simulink model "flightControlSystem"  (R2022b)
settings: Solver=ode3  StartTime=0  StopTime=TFinal  FixedStep=Ts  RelTol=1e-3  EnableMultiTasking=on
undefined symbols (not defined in the file): codertarget, Controller, DiscIntNeverNeededParam, Discrete, Estimator, g, init, orient_ref, pos_ref, Sensors, Time, Ts, var_acc_angle_N, var_bias_gyr_N, var_gyro_p_N, Vehicle
libraries: simulink x52, matrix_library x15, slpidlib x4, ctrlSharedLib x4, sharedtransform x3, visiontransforms x2, dspindex x2, visiontextngfix x1, visionanalysis x1, visionstatistics x1, parrotlib x1
(part 3 of 3)

== system flightControlSystem/Control System/State Estimator/XY Position Estimator/EstimatorVelocity/xy velocity w//o angular velocity compensation ==
  note: Optical flow raw readings are converted to velocity in m/s based on the estimated altitude
  optical_flow : Inport
  z_estimate : Inport  Port=2
  " " : Product  Inputs=**
  Compare To Constant : simulink/Logic and Bit Operations/Compare To Constant  relop=<  const=200*4  OutDataTypeStr=boolean
  Counter Free-Running : simulink/Sources/Counter Free-Running  NumBits=32  tsamp=-1
  Gain : Gain  Gain=-1
  Select dxy : Selector  InputPortWidth=3  IndexOptions=Index vector (dialog)  Indices=[1 2]  OutputSizes=1
  Switch : Switch  Criteria=u2 > Threshold  SaturateOnIntegerOverflow=off  InputSameDT=off
  opticalFlowErrorCorrect : Gain  Gain=1.15
  optical_flow_dx_dy : Outport
  wires:
  Select dxy/1 -> optical_flow_dx_dy/1  "optical_flow_dx_dy"
  " "/1 -> opticalFlowErrorCorrect/1
  opticalFlowErrorCorrect/1 -> Switch/3
  Gain/1 -> " "/2
  Switch/1 -> Select dxy/1
  Counter Free-Running/1 -> Compare To Constant/1
  Compare To Constant/1 -> Switch/2
  optical_flow/1 -> " "/1, Switch/1
  z_estimate/1 -> Gain/1

== matlab function flightControlSystem/Control System/Controller/Position Controller/Position error transformation (Earth to Body frame) ==
  data: yaw input; xy_err_earth input; xy_err_body output
function xy_err_body = fcn(yaw,xy_err_earth)

transformation = [cos(yaw), sin(yaw); -sin(yaw),  cos(yaw)];
xy_err_body = transformation * xy_err_earth;


end

== matlab function flightControlSystem/Image Processing System/Find Angle of a Turn ==
  data: lines input; alpha output; right input; left input
function alpha = getAlpha(lines, right, left)
if right==1 || left==1
    if lines
        %lines(1,1) -- point1.col
        %lines(1,2) -- point1.row
        %lines(1,3) -- point2.col
        %lines(1,4) -- point2.row
        l = double(abs(lines(1,3)-lines(1,1)));
        d = sqrt(double((lines(1,1)-lines(1,3))^2+(lines(1,2)-lines(1,4))^2));
        alpha = acos(l/d);
        
        %Ignore short edge
        if d >= 20
            if right==1
                if (lines(1,2) > lines(1,4) && lines(1,1) <= lines(1,3))||(lines(1,2) < lines(1,4) && lines(1,1) > lines(1,3))
                    alpha = -alpha;
                end
            else
                if (lines(1,2) < lines(1,4) && lines(1,1) <= lines(1,3))||(lines(1,2) > lines(1,4) && lines(1,1) > lines(1,3))
                    alpha = -alpha;
                end
            end
    
            alpha = pi/2 + alpha;
        else
            alpha = 0;
        end
    else
        alpha = 0;
    end
else
    alpha = 0;
end

== stateflow chart flightControlSystem/Control System/Path Planning/Chart ==
  state AlignRight
    during:
    xOut = xOut - 0.0005*sin(yaw_est);
    yOut = yOut + 0.0005*cos(yaw_est);
  state AlignLeft
    during:
    xOut = xOut + 0.0005*sin(yaw_est);
    yOut = yOut - 0.0005*cos(yaw_est);
  state MoveToTargetYawRight
    entry:
    doState = 0;
    during:
    if (doState==0)
    xOut = xOut + distance*cos(yaw_est);
    yOut = yOut + distance*sin(yaw_est);
    yawOut = yaw_est + alpha;
    doState = doState + 1;
    end
  note: Better seperate acute and obtuse, because time for rotating is diff
  state YawRightIni
    during:
    yawOut = yawOut + 0.001;
  note: Ahihi Do Ngok
  state TakeOff
    during:
    xOut = 0;
    yOut = 0;
    zOut = -1.1;
    yawOut = 0;
  state MoveForward
    during:
    xOut = xOut + 0.0005*cos(yaw_est);
    yOut = yOut + 0.0005*sin(yaw_est);
  state YawObtuseLeft
    entry:
    doState = 0;
    during:
    if (doState==0)
    xOut = xOut + distance*cos(yaw_est);
    yOut = yOut + distance*sin(yaw_est);
    yawOut = yaw_est - alpha;
    doState = doState + 1;
    end
  state YawLeftIni
    during:
    yawOut = yawOut - 0.001;
  state EndLineDetected
    during:
    xOut = xOut + 0.0003*cos(yaw_est);
    yOut = yOut + 0.0003*sin(yaw_est);
  state Land
    during:
    zOut = 0
  MoveForward -> AlignRight [order 4] : [(ObtuseRight==1||AcuteRight==1)&&(alpha<pi/18||alpha>17*pi/18)]
  AlignRight -> MoveForward : [up==1]
  AlignLeft -> MoveForward : [up==1]
  MoveForward -> AlignLeft [order 5] : [(ObtuseLeft==1||AcuteLeft==1)&&(alpha<pi/18||alpha>17*pi/18)]
  MoveForward -> MoveToTargetYawRight [order 1] : [(ObtuseRight==1||AcuteRight==1)&&alpha>pi/18&&alpha<17*pi/18]
  MoveToTargetYawRight -> MoveForward : [after(4.5,sec)]
  YawRightIni -> MoveForward : [IniRight==0&&up==1]
  TakeOff -> YawRightIni [order 2] : [after(3,sec)&&IniRight==1]
  (default) -> TakeOff
  TakeOff -> MoveForward [order 1] : [after(3,sec)&&up==1]
  YawObtuseLeft -> MoveForward : [after(4.5,sec)]
  MoveForward -> YawObtuseLeft [order 2] : [(ObtuseLeft==1||AcuteLeft==1)&&alpha>pi/18&&alpha<17*pi/18]
  YawLeftIni -> MoveForward : [IniLeft==0&&up==1]
  MoveForward -> EndLineDetected [order 3] : [up==0&&(ObtuseLeft==0&AcuteLeft==0&ObtuseRight==0&AcuteRight==0)]
  TakeOff -> YawLeftIni [order 3] : [after(3,sec)&&IniLeft==1]
  EndLineDetected -> Land : [circle==1]
  data: circle input; yawOut output single; yaw_est input; ObtuseRight input; AcuteRight input; ObtuseLeft input; AcuteLeft input; distance input; alpha input; up input; doState local; xOut output single; yOut output single; zOut output single; IniLeft input; IniRight input

== matlab function flightControlSystem/Image Processing System/Get Distance to Turning Point from break point ==
  data: distance output; alpha input
function distance = getDistanceToTurn(alpha)

w_path = 0.1;
%Drone position: it's probably not exact at (W/2,H/2), existing a small dis
%between W/2,H/2 and the position
%Dis from drone position (including the deviation) --> break point 
%with z = -1.1
offset = 0.1205;
if alpha > pi/2
    distance = w_path*(tan(alpha-pi/2)+1/cos(alpha-pi/2)) + offset;
else
    beta = pi/2-alpha;
    distance = offset - tan(pi/4-beta/2)*w_path/2;
end
if distance > 1
    distance = 0;
end

== matlab function flightControlSystem/Image Processing System/MATLAB Function ==
  data: R input; G input; BW output; B input
function BW = createMask(R,G,B)

% Define thresholds for channel 1 based on histogram settings
channel1Min = 0.000;
channel1Max = 255.000;

% Define thresholds for channel 2 based on histogram settings
channel2Min = 0.000;
channel2Max = 0.000;

% Define thresholds for channel 3 based on histogram settings
channel3Min = 0.000;
channel3Max = 255.000;

% Create mask based on chosen histogram thresholds
sliderBW = (R >= channel1Min ) & (R <= channel1Max) & ...
    (G >= channel2Min ) & (G <= channel2Max) & ...
    (B >= channel3Min ) & (B <= channel3Max);

BW = sliderBW;
